simulink model "initial_setup"  (R2012b)
settings: Solver=FixedStepDiscrete  StartTime=0.0  StopTime=inf  FixedStep=sample_time  RelTol=1e-3
InitFcn:
  | init_initial_setup;
values from neighbouring files (symbols this model uses):
  fcut_unwrap = 50    [init_initial_setup.m]
  fcut_velocity = 100    [init_initial_setup.m]
  sample_time = 1/update_freq    (= 0.001)    [init_initial_setup.m]
undefined symbols (not defined in the file or in its folder): A_angle_h, A_angle_k, A_angle_lat, angle_midpoint_h, angle_midpoint_k, angle_midpoint_lat, BOOM_MAX_ENCODER_TICKS, BOOM_PITCH_CAL_VALUE_RAD, BOOM_PITCH_CAL_VALUE_TICKS, BOOM_PITCH_ENCODER_RAD_PER_TICK, BOOM_ROLL_CAL_VALUE_RAD, BOOM_ROLL_CAL_VALUE_TICKS, BOOM_ROLL_ENCODER_RAD_PER_TICK, BOOM_YAW_ENCODER_RAD_PER_TICK, control_start_time, HIP_ABS_ENCODER_RAD_PER_TICK, HIP_INC_ENCODER_RAD_PER_TICK, HIP_INC_MAX_ENCODER_TICKS, k_leg_spring, kd_h_sine_walk, kd_k_sine_walk, kd_lat, kd_sea_position, kd_sea_torque, kd_velocity, kp_h_sine_walk, kp_k_sine_walk, kp_lat, kp_sea_position, kp_sea_torque, kp_velocity, LEFT_HIP_CALIB_POS, LEFT_HIP_CALIB_VAL, LEFT_MOTOR_HIP_DIRECTION, LEG1_LEG_A_CALIB_VAL, LEG1_LEG_A_RAD_PER_CNT, LEG1_LEG_B_CALIB_VAL, LEG1_LEG_B_RAD_PER_CNT, LEG1_MOTOR_A_DIRECTION, LEG1_MOTOR_B_DIRECTION, LEG1_TRAN_A_CALIB_VAL, LEG1_TRAN_A_RAD_PER_CNT, LEG1_TRAN_B_CALIB_VAL, LEG1_TRAN_B_RAD_PER_CNT, LEG2_LEG_A_CALIB_VAL, LEG2_LEG_A_RAD_PER_CNT, LEG2_LEG_B_CALIB_VAL, LEG2_LEG_B_RAD_PER_CNT, LEG2_MOTOR_A_DIRECTION, LEG2_MOTOR_B_DIRECTION, LEG2_TRAN_A_CALIB_VAL, LEG2_TRAN_A_RAD_PER_CNT, LEG2_TRAN_B_CALIB_VAL, LEG2_TRAN_B_RAD_PER_CNT, LEG_A_CALIB_LOC, LEG_B_CALIB_LOC, LEG_MTR_GEAR_RATIO, LEG_MTR_MAX_TORQUE, LEG_MTR_MAX_VELOCITY, MTR_HIP_MAX_CURRENT ... (+10)
libraries: xpcethercatlib x160, simulink x34, dspswit3 x1
(part 1 of 4)
settings Model: xpc_rtwmakecfg_data=_xpcethercatlib_  BufferReuse=off  Creator=wmartin  LastModifiedBy=wmartin
settings DataIOCC: MaxDataPoints=1000000000  SaveFormat=StructureWithTime
settings OptimizationCC: BlockReduction=off  OptimizeBlockIOStorage=off  BufferReuse=off  ExpressionFolding=off  LocalBlockOutputs=off
settings HardwareCC: ProdIntDivRoundTo=Zero  ProdEndianess=LittleEndian  ProdHWDeviceType=Generic->32-bit x86 compatible
settings RTWCC: SystemTargetFile=xpctarget.tlc  TemplateMakefile=xpc_default_tmf  Description=xPC Target  RTWVerbose=off  ProcessScript=xpctarget_make_rtw_hook  RTWCompilerOptimization=On
settings xpcTargetCC: TargetFcnLib=ansi_tfl_table_tmw.mat  CodeReplacementLibrary=XPC_BLAS  ParMdlRefBuildCompliant=on  ConcurrentExecutionCompliant=on  CombineSignalStateStructs=off  GRTInterface=on  RL32LogBufSizeModifier=100000000  xPCTaskExecutionProfile=off  xPCRL32EventNumber=5000  xPCLoadParamSetFile=off  xPCConcurrentTasks=off  xPCEnableSFAnimation=off

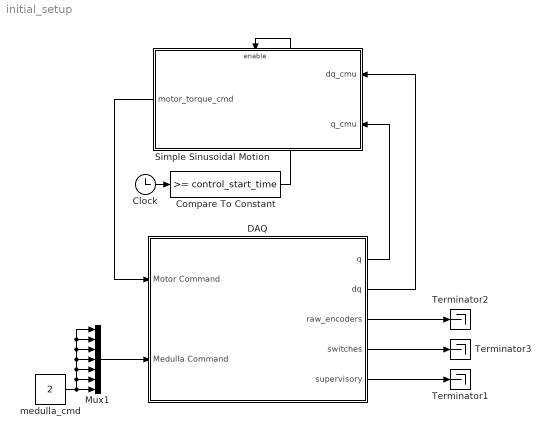
== system initial_setup ==
  Clock : Clock
  Compare To Constant : simulink/Logic and Bit Operations/Compare To Constant  relop=>=  const=control_start_time  OutDataTypeStr=boolean
  DAQ : Subsystem
  Mux1 : Mux  Inputs=7
  Simple Sinusoidal Motion : Subsystem
  Terminator1 : Terminator
  Terminator2 : Terminator
  Terminator3 : Terminator
  medulla_cmd : Constant  Value=2
  wires:
  Mux1/1 -> DAQ/2(Medulla Command)
  DAQ/5(supervisory) -> Terminator1/1
  DAQ/3(raw_encoders) -> Terminator2/1
  DAQ/4(switches) -> Terminator3/1
  Simple Sinusoidal Motion/1(motor_torque_cmd) -> DAQ/1(Motor Command)
  DAQ/1(q) -> Simple Sinusoidal Motion/2(q_cmu)
  DAQ/2(dq) -> Simple Sinusoidal Motion/1(dq_cmu)
  Clock/1 -> Compare To Constant/1
  Compare To Constant/1 -> Simple Sinusoidal Motion/Enable
  medulla_cmd/1 -> Mux1/7, Mux1/1, Mux1/2, Mux1/3, Mux1/4, Mux1/5, Mux1/6

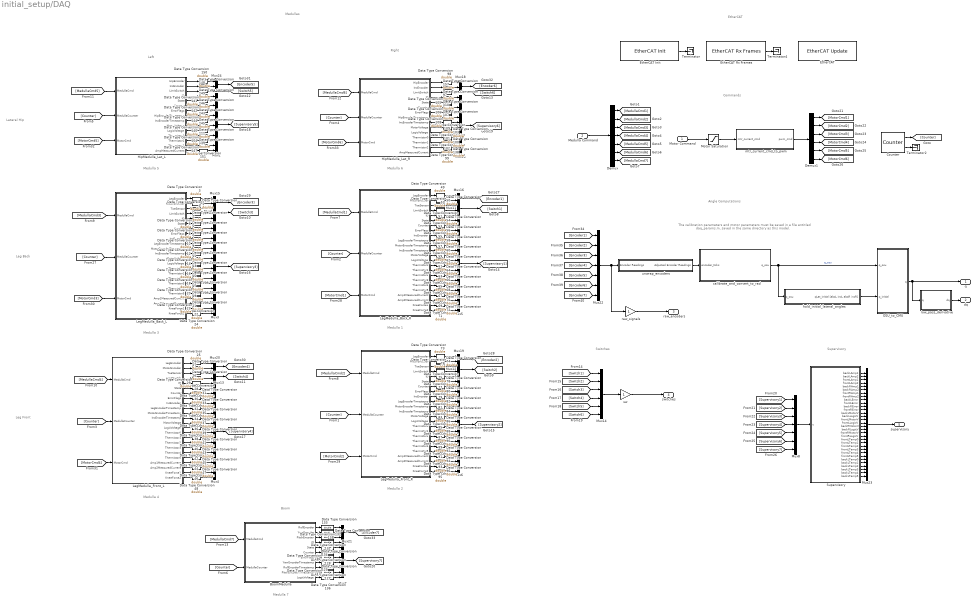
== system initial_setup/DAQ ==
  note: Left
  note: The calibration parameters and motor parameters
      | must be saved in a file entitled daq_params.m, saved in the same directory
      | as this model.
  note: Right
  note: Lateral Hip
  note: Leg Back
  note: Leg Front
  note: Boom
  note: Medullas
  note: EtherCAT
  note: Angle Computations
  note: Commands
  note: Switches
  note: Supervisory
  note: Medulla 1
  note: Medulla 2
  note: Medulla 4
  note: Medulla 3
  note: Medulla 5
  note: Medulla 6
  note: Medulla 7
  Motor Command : Inport
  Medulla Command : Inport  Port=2
  BoomMedulla : Subsystem
  Counter : dspswit3/Counter  Direction=Up  CountEvent=Free running  CounterSize=User defined  MaxCount=65535  InitialCount=0  Output=Count and Hit  HitValue=32  ResetInput=off  SamplesPerFrame=1  Ts=.001  CntDtype=double  HitDtype=Logical
  Data Type Conversion{1..111,127..151,157} (137 alike) : DataTypeConversion  OutDataTypeStr=double
  Demux : Demux  Outputs=7
  Demux1 : Demux  Outputs=6
  EtherCAT : xpcethercatlib/EtherCAT Update   Priority=4  device_id=0  task_id_list=[1]  task_rates=[1]  task_priorities=[1500]
  EtherCAT Init : xpcethercatlib/EtherCAT Init   Priority=0  config_file='atrias_boom.xml'  device_id=0  pci_bus=2  pci_slot=2  enaDC=on  errRptLevel=0  sample_time=-1
  EtherCAT Rx Frames : xpcethercatlib/EtherCAT Rx Frames   Priority=1  device_id=0  sample_time=0
  HipMedulla_Lat_L : Subsystem
  HipMedulla_Lat_R : Subsystem
  LegMedulla_Back_L : Subsystem
  LegMedulla_Back_R : Subsystem
  LegMedulla_Front_L : Subsystem
  LegMedulla_Front_R : Subsystem
  Motor Saturation : Saturate  UpperLimit=60  LowerLimit=-60
  Mux1 : Mux  Inputs=12
  Mux10 : Mux  Inputs=12
  Mux{2,11..13,15..16,18..20,24} (10 alike) : Mux  Inputs=2
  Mux14 : Mux  Inputs=6
  Mux21 : Mux  Inputs=3
  Mux22 : Mux  Inputs=7
  Mux23 : Mux  Inputs=32
  Mux{3..6} (4 alike) : Mux  Inputs=20
  Mux7 : Mux  Inputs=8
  Mux8 : Mux  Inputs=7
  OSU_to_CMU : Subsystem
  Supervisory : MATLAB Function  TreatAsAtomicUnit=on
  Terminator : Terminator
  Terminator2 : Terminator
  Terminator4 : Terminator
  calibrate_and_convert_to_rad : Subsystem
  hold_initial_lateral_angles : Subsystem
  low_pass_derivative : Subsystem
  mtr_current_cmd_to_pwm : Subsystem
  raw_signals : Gain
  sw : Gain
  unwrap_encoders : Subsystem
  q : Outport
  dq : Outport  Port=2
  raw_encoders : Outport  Port=3
  switches : Outport  Port=4
  supervisory : Outport  Port=5
  wires:
  EtherCAT Rx Frames/1 -> Terminator4/1
  OSU_to_CMU/1(q) -> q/1, low_pass_derivative/1(q)
  raw_signals/1 -> raw_encoders/1
  BoomMedulla/11(LogicVoltage) -> Data Type Conversion136/1
  BoomMedulla/10(PitchEncoderTimestamp) -> Data Type Conversion137/1
  BoomMedulla/9(RollEncoderTimestamp) -> Data Type Conversion127/1
  BoomMedulla/8(YawEncoderTimestamp) -> Data Type Conversion129/1
  BoomMedulla/7(ErrorFlags) -> Data Type Conversion130/1
  BoomMedulla/6(Counter) -> Data Type Conversion128/1
  BoomMedulla/5(State) -> Data Type Conversion134/1
  BoomMedulla/4(ID) -> Data Type Conversion135/1
  BoomMedulla/3(PitchEncoder) -> Data Type Conversion131/1
  BoomMedulla/2(YawEncoder) -> Data Type Conversion132/1
  BoomMedulla/1(RollEncoder) -> Data Type Conversion133/1
  Data Type Conversion133/1 -> Mux21/1
  Data Type Conversion132/1 -> Mux21/2
  Data Type Conversion131/1 -> Mux21/3
  Data Type Conversion135/1 -> Mux7/1
  Data Type Conversion134/1 -> Mux7/2
  Data Type Conversion128/1 -> Mux7/3
  Data Type Conversion130/1 -> Mux7/4
  Data Type Conversion129/1 -> Mux7/5
  Data Type Conversion127/1 -> Mux7/6
  Data Type Conversion137/1 -> Mux7/7
  Data Type Conversion136/1 -> Mux7/8
  HipMedulla_Lat_R/15(AmpMeasuredCurrent) -> Data Type Conversion138/1
  HipMedulla_Lat_R/14(Thermistor2) -> Data Type Conversion99/1
  HipMedulla_Lat_R/13(Thermistor1) -> Data Type Conversion100/1
  HipMedulla_Lat_R/12(Thermistor0) -> Data Type Conversion102/1
  HipMedulla_Lat_R/11(LogicVoltage) -> Data Type Conversion103/1
  HipMedulla_Lat_R/10(MotorVoltage) -> Data Type Conversion101/1
  HipMedulla_Lat_R/9(IncEncoderTimestamp) -> Data Type Conversion108/1
  HipMedulla_Lat_R/8(HipEncoderTimestamp) -> Data Type Conversion109/1
  HipMedulla_Lat_R/7(ErrorFlags) -> Data Type Conversion106/1
  HipMedulla_Lat_R/6(Counter) -> Data Type Conversion107/1
  HipMedulla_Lat_R/5(State) -> Data Type Conversion105/1
  HipMedulla_Lat_R/4(ID) -> Data Type Conversion110/1
  HipMedulla_Lat_R/3(LimitSwitch) -> Data Type Conversion157/1
  HipMedulla_Lat_R/2(IncEncoder) -> Data Type Conversion97/1
  HipMedulla_Lat_R/1(HipEncoder) -> Data Type Conversion98/1
  Data Type Conversion98/1 -> Mux18/1
  Data Type Conversion97/1 -> Mux18/2
  Data Type Conversion110/1 -> Mux10/1
  Data Type Conversion105/1 -> Mux10/2
  Data Type Conversion107/1 -> Mux10/3
  Data Type Conversion106/1 -> Mux10/4
  Data Type Conversion109/1 -> Mux10/5
  Data Type Conversion108/1 -> Mux10/6
  Data Type Conversion101/1 -> Mux10/7
  Data Type Conversion103/1 -> Mux10/8
  Data Type Conversion102/1 -> Mux10/9
  Data Type Conversion100/1 -> Mux10/10
  Data Type Conversion99/1 -> Mux10/11
  mtr_current_cmd_to_pwm/1(pwm_cmd) -> Demux1/1
  Data Type Conversion50/1 -> Mux16/2
  Data Type Conversion49/1 -> Mux16/1
  Data Type Conversion48/1 -> Mux4/20
  Data Type Conversion47/1 -> Mux4/19
  Data Type Conversion46/1 -> Mux4/18
  Data Type Conversion45/1 -> Mux4/17
  Data Type Conversion44/1 -> Mux4/16
  Data Type Conversion43/1 -> Mux4/15
  Data Type Conversion42/1 -> Mux4/14
  Data Type Conversion41/1 -> Mux4/13
  Data Type Conversion40/1 -> Mux4/12
  Data Type Conversion39/1 -> Mux4/11
  Data Type Conversion38/1 -> Mux4/10
  Data Type Conversion37/1 -> Mux4/9
  Data Type Conversion36/1 -> Mux4/8
  Data Type Conversion35/1 -> Mux4/7
  Data Type Conversion34/1 -> Mux4/6
  Data Type Conversion33/1 -> Mux4/5
  Data Type Conversion32/1 -> Mux4/4
  Data Type Conversion31/1 -> Mux4/3
  Data Type Conversion30/1 -> Mux4/2
  Data Type Conversion29/1 -> Mux4/1
  Data Type Conversion28/1 -> Mux13/2
  Data Type Conversion27/1 -> Mux13/1
  Data Type Conversion26/1 -> Mux20/2
  Data Type Conversion25/1 -> Mux20/1
  Data Type Conversion24/1 -> Mux3/20
  Data Type Conversion23/1 -> Mux3/19
  Data Type Conversion22/1 -> Mux3/18
  Data Type Conversion21/1 -> Mux3/17
  Data Type Conversion20/1 -> Mux3/16
  Data Type Conversion19/1 -> Mux3/15
  Data Type Conversion18/1 -> Mux3/14
  Data Type Conversion17/1 -> Mux3/13
  Data Type Conversion16/1 -> Mux3/12
  Data Type Conversion15/1 -> Mux3/11
  Data Type Conversion14/1 -> Mux3/10
  Data Type Conversion13/1 -> Mux3/9
  Data Type Conversion12/1 -> Mux3/8
  Data Type Conversion11/1 -> Mux3/7
  Data Type Conversion10/1 -> Mux3/6
  Data Type Conversion9/1 -> Mux3/5
  Data Type Conversion8/1 -> Mux3/4
  Data Type Conversion7/1 -> Mux3/3
  Data Type Conversion6/1 -> Mux3/2
  Data Type Conversion5/1 -> Mux3/1
  Data Type Conversion4/1 -> Mux2/2
  Data Type Conversion2/1 -> Mux2/1
  Data Type Conversion1/1 -> Mux15/2
  Data Type Conversion3/1 -> Mux15/1
  LegMedulla_Back_R/1(LegEncoder) -> Data Type Conversion49/1
  LegMedulla_Back_L/1(LegEncoder) -> Data Type Conversion3/1
  LegMedulla_Back_R/2(MotorEncoder) -> Data Type Conversion50/1
  Motor Saturation/1 -> mtr_current_cmd_to_pwm/1(mtr_current_cmd)
  Motor Command/1 -> Motor Saturation/1
  Data Type Conversion138/1 -> Mux10/12
  Data Type Conversion96/1 -> Mux6/20
  Data Type Conversion95/1 -> Mux6/19
  Data Type Conversion94/1 -> Mux6/18
  Data Type Conversion93/1 -> Mux6/17
  Data Type Conversion92/1 -> Mux6/16
  Data Type Conversion91/1 -> Mux6/15
  Data Type Conversion90/1 -> Mux6/14
  Data Type Conversion89/1 -> Mux6/13
  Data Type Conversion88/1 -> Mux6/12
  Data Type Conversion87/1 -> Mux6/11
  Data Type Conversion86/1 -> Mux6/10
  Data Type Conversion85/1 -> Mux6/9
  Data Type Conversion84/1 -> Mux6/8
  Data Type Conversion83/1 -> Mux6/7
  Data Type Conversion82/1 -> Mux6/6
  Data Type Conversion81/1 -> Mux6/5
  Data Type Conversion80/1 -> Mux6/4
  Data Type Conversion79/1 -> Mux6/3
  Data Type Conversion78/1 -> Mux6/2
  Data Type Conversion77/1 -> Mux6/1
  Data Type Conversion76/1 -> Mux12/2
  Data Type Conversion75/1 -> Mux12/1
  Data Type Conversion74/1 -> Mux19/2
  Data Type Conversion73/1 -> Mux19/1
  Data Type Conversion72/1 -> Mux5/20
  Data Type Conversion71/1 -> Mux5/19
  Data Type Conversion70/1 -> Mux5/18
  Data Type Conversion69/1 -> Mux5/17
  Data Type Conversion68/1 -> Mux5/16
  Data Type Conversion67/1 -> Mux5/15
  Data Type Conversion66/1 -> Mux5/14
  Data Type Conversion65/1 -> Mux5/13
  Data Type Conversion64/1 -> Mux5/12
  Data Type Conversion63/1 -> Mux5/11
  Data Type Conversion62/1 -> Mux5/10
  Data Type Conversion61/1 -> Mux5/9
  Data Type Conversion60/1 -> Mux5/8
  Data Type Conversion59/1 -> Mux5/7
  Data Type Conversion58/1 -> Mux5/6
  Data Type Conversion57/1 -> Mux5/5
  Data Type Conversion56/1 -> Mux5/4
  Data Type Conversion55/1 -> Mux5/3
  Data Type Conversion54/1 -> Mux5/2
  Data Type Conversion53/1 -> Mux5/1
  Data Type Conversion52/1 -> Mux11/2
  Data Type Conversion51/1 -> Mux11/1
  LegMedulla_Front_R/3(ToeSensor) -> Data Type Conversion75/1
  LegMedulla_Front_R/2(MotorEncoder) -> Data Type Conversion74/1
  LegMedulla_Front_R/1(LegEncoder) -> Data Type Conversion73/1
  Counter/2 -> Terminator2/1
  EtherCAT Init/1 -> Terminator/1
  Medulla Command/1 -> Demux/1
  LegMedulla_Front_R/24(KneeForce2) -> Data Type Conversion96/1
  LegMedulla_Back_R/24(KneeForce2) -> Data Type Conversion72/1
  LegMedulla_Front_R/23(KneeForce1) -> Data Type Conversion95/1
  LegMedulla_Front_R/22(Amp2MeasuredCurrent) -> Data Type Conversion94/1
  LegMedulla_Front_R/21(Amp1MeasuredCurrent) -> Data Type Conversion93/1
  LegMedulla_Front_R/20(Thermistor5) -> Data Type Conversion92/1
  LegMedulla_Front_R/19(Thermistor4) -> Data Type Conversion91/1
  LegMedulla_Front_R/18(Thermistor3) -> Data Type Conversion90/1
  LegMedulla_Front_R/17(Thermistor2) -> Data Type Conversion89/1
  LegMedulla_Front_R/16(Thermistor1) -> Data Type Conversion88/1
  LegMedulla_Front_R/15(Thermistor0) -> Data Type Conversion87/1
  LegMedulla_Front_R/14(LogicVoltage) -> Data Type Conversion86/1
  LegMedulla_Front_R/13(MotorVoltage) -> Data Type Conversion85/1
  LegMedulla_Front_R/12(IncEncoderTimestamp) -> Data Type Conversion84/1
  LegMedulla_Front_R/11(MotorEncoderTimestamp) -> Data Type Conversion83/1
  LegMedulla_Front_R/10(LegEncoderTimestamp) -> Data Type Conversion82/1
  LegMedulla_Front_R/9(IncEncoder) -> Data Type Conversion81/1
  LegMedulla_Front_R/8(ErrorFlags) -> Data Type Conversion80/1
  LegMedulla_Front_R/7(Counter) -> Data Type Conversion79/1
  LegMedulla_Front_R/6(State) -> Data Type Conversion78/1
  LegMedulla_Front_R/5(ID) -> Data Type Conversion77/1
  LegMedulla_Front_R/4(LimitSwitch) -> Data Type Conversion76/1
  LegMedulla_Back_R/23(KneeForce1) -> Data Type Conversion71/1
  LegMedulla_Back_R/22(Amp2MeasuredCurrent) -> Data Type Conversion70/1
  LegMedulla_Back_R/21(Amp1MeasuredCurrent) -> Data Type Conversion69/1
  LegMedulla_Back_R/20(Thermistor5) -> Data Type Conversion68/1
  LegMedulla_Back_R/19(Thermistor4) -> Data Type Conversion67/1
  LegMedulla_Back_R/18(Thermistor3) -> Data Type Conversion66/1
  LegMedulla_Back_R/17(Thermistor2) -> Data Type Conversion65/1
  LegMedulla_Back_R/16(Thermistor1) -> Data Type Conversion64/1
  LegMedulla_Back_R/15(Thermistor0) -> Data Type Conversion63/1
  LegMedulla_Back_R/14(LogicVoltage) -> Data Type Conversion62/1
  LegMedulla_Back_R/13(MotorVoltage) -> Data Type Conversion61/1
  LegMedulla_Back_R/12(IncEncoderTimestamp) -> Data Type Conversion60/1
  LegMedulla_Back_R/11(MotorEncoderTimestamp) -> Data Type Conversion59/1
  LegMedulla_Back_R/10(LegEncoderTimestamp) -> Data Type Conversion58/1
  LegMedulla_Back_R/9(IncEncoder) -> Data Type Conversion57/1
  LegMedulla_Back_R/8(ErrorFlags) -> Data Type Conversion56/1
  LegMedulla_Back_R/7(Counter) -> Data Type Conversion55/1
  LegMedulla_Back_R/6(State) -> Data Type Conversion54/1
  LegMedulla_Back_R/5(ID) -> Data Type Conversion53/1
  LegMedulla_Back_R/4(LimitSwitch) -> Data Type Conversion52/1
  LegMedulla_Back_R/3(ToeSensor) -> Data Type Conversion51/1
  LegMedulla_Front_L/24(KneeForce2) -> Data Type Conversion48/1
  LegMedulla_Back_L/24(KneeForce2) -> Data Type Conversion24/1
  LegMedulla_Front_L/23(KneeForce1) -> Data Type Conversion47/1
  LegMedulla_Front_L/22(Amp2MeasuredCurrent) -> Data Type Conversion46/1
  LegMedulla_Front_L/21(Amp1MeasuredCurrent) -> Data Type Conversion45/1
  LegMedulla_Front_L/20(Thermistor5) -> Data Type Conversion44/1
  LegMedulla_Front_L/19(Thermistor4) -> Data Type Conversion43/1
  LegMedulla_Front_L/18(Thermistor3) -> Data Type Conversion42/1
  LegMedulla_Front_L/17(Thermistor2) -> Data Type Conversion41/1
  LegMedulla_Front_L/16(Thermistor1) -> Data Type Conversion40/1
  LegMedulla_Front_L/15(Thermistor0) -> Data Type Conversion39/1
  LegMedulla_Front_L/14(LogicVoltage) -> Data Type Conversion38/1
  LegMedulla_Front_L/13(MotorVoltage) -> Data Type Conversion37/1
  LegMedulla_Front_L/12(IncEncoderTimestamp) -> Data Type Conversion36/1
  LegMedulla_Front_L/11(MotorEncoderTimestamp) -> Data Type Conversion35/1
  LegMedulla_Front_L/10(LegEncoderTimestamp) -> Data Type Conversion34/1
  LegMedulla_Front_L/9(IncEncoder) -> Data Type Conversion33/1
  LegMedulla_Front_L/8(ErrorFlags) -> Data Type Conversion32/1
  LegMedulla_Front_L/7(Counter) -> Data Type Conversion31/1
  LegMedulla_Front_L/6(State) -> Data Type Conversion30/1
  LegMedulla_Front_L/5(ID) -> Data Type Conversion29/1
  LegMedulla_Front_L/4(LimitSwitch) -> Data Type Conversion28/1
  LegMedulla_Front_L/3(ToeSensor) -> Data Type Conversion27/1
  LegMedulla_Front_L/2(MotorEncoder) -> Data Type Conversion26/1
  LegMedulla_Front_L/1(LegEncoder) -> Data Type Conversion25/1
  LegMedulla_Back_L/23(KneeForce1) -> Data Type Conversion23/1
  LegMedulla_Back_L/22(Amp2MeasuredCurrent) -> Data Type Conversion22/1
  LegMedulla_Back_L/21(Amp1MeasuredCurrent) -> Data Type Conversion21/1
  LegMedulla_Back_L/20(Thermistor5) -> Data Type Conversion20/1
  LegMedulla_Back_L/19(Thermistor4) -> Data Type Conversion19/1
  LegMedulla_Back_L/18(Thermistor3) -> Data Type Conversion18/1
  LegMedulla_Back_L/17(Thermistor2) -> Data Type Conversion17/1
  LegMedulla_Back_L/16(Thermistor1) -> Data Type Conversion16/1
  LegMedulla_Back_L/15(Thermistor0) -> Data Type Conversion15/1
  LegMedulla_Back_L/14(LogicVoltage) -> Data Type Conversion14/1
  LegMedulla_Back_L/13(MotorVoltage) -> Data Type Conversion13/1
  LegMedulla_Back_L/12(IncEncoderTimestamp) -> Data Type Conversion12/1
  LegMedulla_Back_L/11(MotorEncoderTimestamp) -> Data Type Conversion11/1
  LegMedulla_Back_L/10(LegEncoderTimestamp) -> Data Type Conversion10/1
  LegMedulla_Back_L/9(IncEncoder) -> Data Type Conversion9/1
  LegMedulla_Back_L/8(ErrorFlags) -> Data Type Conversion8/1
  LegMedulla_Back_L/7(Counter) -> Data Type Conversion7/1
  LegMedulla_Back_L/6(State) -> Data Type Conversion6/1
  LegMedulla_Back_L/5(ID) -> Data Type Conversion5/1
  LegMedulla_Back_L/4(LimitSwitch) -> Data Type Conversion4/1
  LegMedulla_Back_L/3(ToeSensor) -> Data Type Conversion2/1
  LegMedulla_Back_L/2(MotorEncoder) -> Data Type Conversion1/1
  Counter/1 -> [Counter]
  [Counter] -> LegMedulla_Back_L/2(MedullaCounter)
  [Counter] -> LegMedulla_Front_L/2(MedullaCounter)
  [Counter] -> LegMedulla_Back_R/2(MedullaCounter)
  [Counter] -> LegMedulla_Front_R/2(MedullaCounter)
  [Counter] -> HipMedulla_Lat_R/2(MedullaCounter)
  [Counter] -> HipMedulla_Lat_L/2(MedullaCounter)
  [Counter] -> BoomMedulla/2(MedullaCounter)
  Demux/2 -> [MedullaCmd2]
  Demux/1 -> [MedullaCmd1]
  Demux/3 -> [MedullaCmd3]
  Demux/4 -> [MedullaCmd4]
  Demux/5 -> [MedullaCmd5]
  Demux/6 -> [MedullaCmd6]
  Demux/7 -> [MedullaCmd7]
  [MedullaCmd3] -> LegMedulla_Back_L/1(MedullaCmd)
  [MedullaCmd4] -> LegMedulla_Front_L/1(MedullaCmd)
  [MedullaCmd1] -> LegMedulla_Back_R/1(MedullaCmd)
  [MedullaCmd2] -> LegMedulla_Front_R/1(MedullaCmd)
  [MedullaCmd6] -> HipMedulla_Lat_R/1(MedullaCmd)
  [MedullaCmd7] -> BoomMedulla/1(MedullaCmd)
  [MedullaCmd5] -> HipMedulla_Lat_L/1(MedullaCmd)
  Data Type Conversion157/1 -> [Switch6]
  [Switch1] -> Mux14/1
  [Switch2] -> Mux14/2
  [Switch3] -> Mux14/3
  [Switch4] -> Mux14/4
  [Switch5] -> Mux14/5
  [Switch6] -> Mux14/6
  sw/1 -> switches/1
  low_pass_derivative/1(dq) -> dq/1
  calibrate_and_convert_to_rad/1(q_osu) -> hold_initial_lateral_angles/1(q_osu), OSU_to_CMU/1(q_osu)  "q_osu"
  hold_initial_lateral_angles/1(qLat_initial [absL incL absR incR]) -> OSU_to_CMU/2(q_initial)
  unwrap_encoders/1(Adjusted Encoder Readings) -> calibrate_and_convert_to_rad/1(encoder_ticks)
  [MotorCmd3] -> LegMedulla_Back_L/3(MotorCmd)
  [MotorCmd4] -> LegMedulla_Front_L/3(MotorCmd)
  [MotorCmd1] -> LegMedulla_Back_R/3(MotorCmd)
  [MotorCmd2] -> LegMedulla_Front_R/3(MotorCmd)
  [MotorCmd6] -> HipMedulla_Lat_R/3(MotorCmd)
  [MotorCmd5] -> HipMedulla_Lat_L/3(MotorCmd)
  Demux1/1 -> [MotorCmd1]
  Demux1/2 -> [MotorCmd2]
  Demux1/3 -> [MotorCmd3]
  Demux1/4 -> [MotorCmd4]
  Demux1/5 -> [MotorCmd5]
  Demux1/6 -> [MotorCmd6]
  Mux2/1 -> [Switch3]
  Mux3/1 -> [Supervisory3]
  Mux4/1 -> [Supervisory4]
  Mux5/1 -> [Supervisory1]
  Mux6/1 -> [Supervisory2]
  Mux7/1 -> [Supervisory7]
  [Supervisory1] -> Mux8/1
  [Supervisory2] -> Mux8/2
  [Supervisory3] -> Mux8/3
  [Supervisory4] -> Mux8/4
  [Supervisory5] -> Mux8/5
  [Supervisory6] -> Mux8/6
  [Supervisory7] -> Mux8/7
  Mux8/1 -> Supervisory/1(u)
  Mux10/1 -> [Supervisory6]
  Mux11/1 -> [Switch1]
  Mux12/1 -> [Switch2]
  Mux13/1 -> [Switch4]
  Mux14/1 -> sw/1
  Mux15/1 -> [Encoder3]
  Mux16/1 -> [Encoder1]
  Mux18/1 -> [Encoder6]
  Mux19/1 -> [Encoder2]
  Mux20/1 -> [Encoder4]
  Mux21/1 -> [Encoder7]
  [Encoder7] -> Mux22/7
  [Encoder6] -> Mux22/6
  [Encoder5] -> Mux22/5
  [Encoder4] -> Mux22/4
  [Encoder3] -> Mux22/3
  [Encoder2] -> Mux22/2
  [Encoder1] -> Mux22/1
  Mux22/1 -> raw_signals/1, unwrap_encoders/1(Encoder Readings)
  Supervisory/1(backLAmp1) -> Mux23/1
  Supervisory/2(backLAmp2) -> Mux23/2
  Supervisory/3(frontLAmp1) -> Mux23/3
  Supervisory/4(frontLAmp2) -> Mux23/4
  Supervisory/5(backRAmp1) -> Mux23/5
  Supervisory/6(backRAmp2) -> Mux23/6
  Supervisory/7(frontRAmp1) -> Mux23/7
  Supervisory/9(backLError) -> Mux23/9
  Supervisory/8(frontRAmp2) -> Mux23/8
  Supervisory/10(frontLError) -> Mux23/10
  Supervisory/11(backRError) -> Mux23/11
  Supervisory/12(frontRError) -> Mux23/12
  Supervisory/13(backLMotorV) -> Mux23/13
  Supervisory/14(backLLogicV) -> Mux23/14
  Supervisory/15(frontLMotorV) -> Mux23/15
  Supervisory/16(frontLLogicV) -> Mux23/16
  Supervisory/17(backRMotorV) -> Mux23/17
  Supervisory/18(backRLogicV) -> Mux23/18
  Supervisory/19(frontRMotorV) -> Mux23/19
  Supervisory/20(frontRLogicV) -> Mux23/20
  Mux23/1 -> supervisory/1
  HipMedulla_Lat_L/15(AmpMeasuredCurrent) -> Data Type Conversion147/1
  HipMedulla_Lat_L/14(Thermistor2) -> Data Type Conversion151/1
  HipMedulla_Lat_L/13(Thermistor1) -> Data Type Conversion104/1
  HipMedulla_Lat_L/12(Thermistor0) -> Data Type Conversion139/1
  HipMedulla_Lat_L/11(LogicVoltage) -> Data Type Conversion140/1
  HipMedulla_Lat_L/10(MotorVoltage) -> Data Type Conversion111/1
  HipMedulla_Lat_L/9(IncEncoderTimestamp) -> Data Type Conversion144/1
  HipMedulla_Lat_L/8(HipEncoderTimestamp) -> Data Type Conversion145/1
  HipMedulla_Lat_L/7(ErrorFlags) -> Data Type Conversion142/1
  HipMedulla_Lat_L/6(Counter) -> Data Type Conversion143/1
  HipMedulla_Lat_L/5(State) -> Data Type Conversion141/1
  HipMedulla_Lat_L/4(ID) -> Data Type Conversion146/1
  HipMedulla_Lat_L/3(LimitSwitch) -> Data Type Conversion148/1
  HipMedulla_Lat_L/2(IncEncoder) -> Data Type Conversion149/1
  HipMedulla_Lat_L/1(HipEncoder) -> Data Type Conversion150/1
  Data Type Conversion150/1 -> Mux24/1
  Data Type Conversion149/1 -> Mux24/2
  Data Type Conversion146/1 -> Mux1/1
  Data Type Conversion141/1 -> Mux1/2
  Data Type Conversion143/1 -> Mux1/3
  Data Type Conversion142/1 -> Mux1/4
  Data Type Conversion145/1 -> Mux1/5
  Data Type Conversion144/1 -> Mux1/6
  Data Type Conversion111/1 -> Mux1/7
  Data Type Conversion140/1 -> Mux1/8
  Data Type Conversion139/1 -> Mux1/9
  Data Type Conversion104/1 -> Mux1/10
  Data Type Conversion151/1 -> Mux1/11
  Data Type Conversion147/1 -> Mux1/12
  Data Type Conversion148/1 -> [Switch5]
  Mux1/1 -> [Supervisory5]
  Mux24/1 -> [Encoder5]
  Supervisory/21(frontLTemp0) -> Mux23/21
  Supervisory/22(frontLTemp1) -> Mux23/22
  Supervisory/23(frontLTemp2) -> Mux23/23
  Supervisory/24(frontLTemp3) -> Mux23/24
  Supervisory/25(frontLTemp4) -> Mux23/25
  Supervisory/26(frontLTemp5) -> Mux23/26
  Supervisory/28(backLTemp1) -> Mux23/28
  Supervisory/27(backLTemp0) -> Mux23/27
  Supervisory/29(backLTemp2) -> Mux23/29
  Supervisory/30(backLTemp3) -> Mux23/30
  Supervisory/31(backLTemp4) -> Mux23/31
  Supervisory/32(backLTemp5) -> Mux23/32

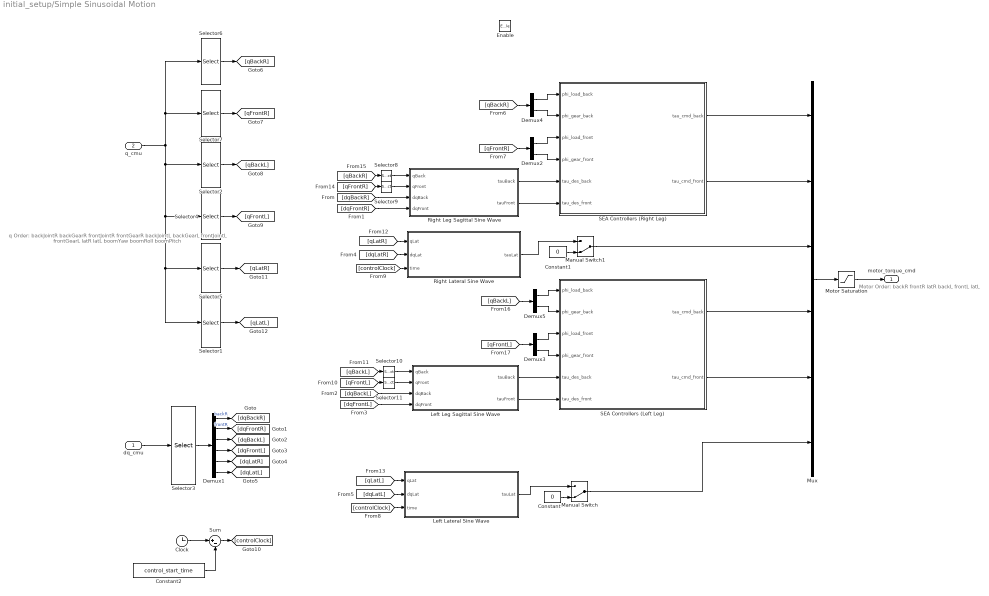
== system initial_setup/Simple Sinusoidal Motion ==
  note: q Order:
      |
      | backJointR
      | backGearR
      | frontJointR
      | frontGearR
      |
      | backJointL
      | backGearL
      | frontJointL
      | frontGearL
      |
      | latR
      | latL
      |
      | boomYaw
      | boomRoll
      | boomPitch
  note: Motor Order:
      |
      | backR
      | frontR
      | latR
      | backL
      | frontL
      | latL
  dq_cmu : Inport
  q_cmu : Inport  Port=2
  Enable : EnablePort  StatesWhenEnabling=reset
  Clock : Clock
  Constant : Constant  Value=0
  Constant1 : Constant  Value=0
  Constant2 : Constant  Value=control_start_time
  Demux1 : Demux  Outputs=6
  Demux{2..5} (4 alike) : Demux  Outputs=2
  Left Lateral Sine Wave : Subsystem
  Left Leg Sagittal Sine Wave : Subsystem
  Manual Switch : ManualSwitch  CurrentSetting=0
  Manual Switch1 : ManualSwitch  CurrentSetting=0
  Motor Saturation : Saturate  UpperLimit=6  LowerLimit=-6
  Mux : Mux  Inputs=6
  Right Lateral Sine Wave : Subsystem
  Right Leg Sagittal Sine Wave : Subsystem
  SEA Controllers (Left Leg) : Subsystem
  SEA Controllers (Right Leg) : Subsystem
  Selector1 : Selector  InputPortWidth=13  IndexOptions=Index vector (dialog)  Indices=[10]  OutputSizes=1
  Selector{8..11} (4 alike) : Selector  InputPortWidth=2  IndexOptions=Index vector (dialog)  Indices=[2]  OutputSizes=1
  Selector2 : Selector  InputPortWidth=13  IndexOptions=Index vector (dialog)  Indices=[5 6]  OutputSizes=1
  Selector3 : Selector  InputPortWidth=13  IndexOptions=Index vector (dialog)  Indices=[2 4 6 8 9 10]  OutputSizes=1
  Selector4 : Selector  InputPortWidth=13  IndexOptions=Index vector (dialog)  Indices=[7 8]  OutputSizes=1
  Selector5 : Selector  InputPortWidth=13  IndexOptions=Index vector (dialog)  Indices=[9]  OutputSizes=1
  Selector6 : Selector  InputPortWidth=13  IndexOptions=Index vector (dialog)  Indices=[1 2]  OutputSizes=1
  Selector7 : Selector  InputPortWidth=13  IndexOptions=Index vector (dialog)  Indices=[3 4]  OutputSizes=1
  Sum : Sum  Inputs=|+-
  motor_torque_cmd : Outport  OutputWhenDisabled=reset  InitialOutput=[0 0 0 0 0 0]
  wires:
  Mux/1 -> Motor Saturation/1
  Motor Saturation/1 -> motor_torque_cmd/1
  dq_cmu/1 -> Selector3/1
  Selector3/1 -> Demux1/1
  Right Lateral Sine Wave/1(tauLat) -> Manual Switch1/1
  Left Lateral Sine Wave/1(tauLat) -> Manual Switch/1
  Manual Switch1/1 -> Mux/3
  Manual Switch/1 -> Mux/6
  Constant/1 -> Manual Switch/2
  Constant1/1 -> Manual Switch1/2
  Clock/1 -> Sum/1
  Constant2/1 -> Sum/2
  [qBackR] -> Demux4/1
  [qFrontR] -> Demux2/1
  Demux2/2 -> SEA Controllers (Right Leg)/4(phi_gear_front)
  Selector5/1 -> [qLatR]
  Selector1/1 -> [qLatL]
  Demux1/1 -> [dqBackR]  "backR"
  [dqBackR] -> Right Leg Sagittal Sine Wave/3(dqBack)
  [dqFrontR] -> Right Leg Sagittal Sine Wave/4(dqFront)
  Demux1/2 -> [dqFrontR]  "frontR"
  Demux1/3 -> [dqBackL]
  Demux1/4 -> [dqFrontL]
  [dqBackL] -> Left Leg Sagittal Sine Wave/3(dqBack)
  [dqFrontL] -> Left Leg Sagittal Sine Wave/4(dqFront)
  Demux1/5 -> [dqLatR]
  Demux1/6 -> [dqLatL]
  [dqLatR] -> Right Lateral Sine Wave/2(dqLat)
  [dqLatL] -> Left Lateral Sine Wave/2(dqLat)
  Selector6/1 -> [qBackR]
  Selector7/1 -> [qFrontR]
  Selector2/1 -> [qBackL]
  Selector4/1 -> [qFrontL]
  Sum/1 -> [controlClock]
  [controlClock] -> Left Lateral Sine Wave/3(time)
  [controlClock] -> Right Lateral Sine Wave/3(time)
  q_cmu/1 -> Selector1/1, Selector5/1, Selector4/1, Selector2/1, Selector7/1, Selector6/1
  [qLatL] -> Left Lateral Sine Wave/1(qLat)
  [qLatR] -> Right Lateral Sine Wave/1(qLat)
  Right Leg Sagittal Sine Wave/1(tauBack) -> SEA Controllers (Right Leg)/5(tau_des_back)
  Right Leg Sagittal Sine Wave/2(tauFront) -> SEA Controllers (Right Leg)/6(tau_des_front)
  Demux2/1 -> SEA Controllers (Right Leg)/3(phi_load_front)
  SEA Controllers (Right Leg)/1(tau_cmd_back) -> Mux/1
  SEA Controllers (Right Leg)/2(tau_cmd_front) -> Mux/2
  [qBackR] -> Selector8/1
  Selector8/1 -> Right Leg Sagittal Sine Wave/1(qBack)
  [qFrontR] -> Selector9/1
  Selector9/1 -> Right Leg Sagittal Sine Wave/2(qFront)
  Demux4/1 -> SEA Controllers (Right Leg)/1(phi_load_back)
  Demux4/2 -> SEA Controllers (Right Leg)/2(phi_gear_back)
  Selector10/1 -> Left Leg Sagittal Sine Wave/1(qBack)
  Selector11/1 -> Left Leg Sagittal Sine Wave/2(qFront)
  [qBackL] -> Selector10/1
  [qFrontL] -> Selector11/1
  SEA Controllers (Left Leg)/1(tau_cmd_back) -> Mux/4
  SEA Controllers (Left Leg)/2(tau_cmd_front) -> Mux/5
  Left Leg Sagittal Sine Wave/1(tauBack) -> SEA Controllers (Left Leg)/5(tau_des_back)
  Left Leg Sagittal Sine Wave/2(tauFront) -> SEA Controllers (Left Leg)/6(tau_des_front)
  [qBackL] -> Demux5/1
  [qFrontL] -> Demux3/1
  Demux3/2 -> SEA Controllers (Left Leg)/4(phi_gear_front)
  Demux3/1 -> SEA Controllers (Left Leg)/3(phi_load_front)
  Demux5/1 -> SEA Controllers (Left Leg)/1(phi_load_back)
  Demux5/2 -> SEA Controllers (Left Leg)/2(phi_gear_back)

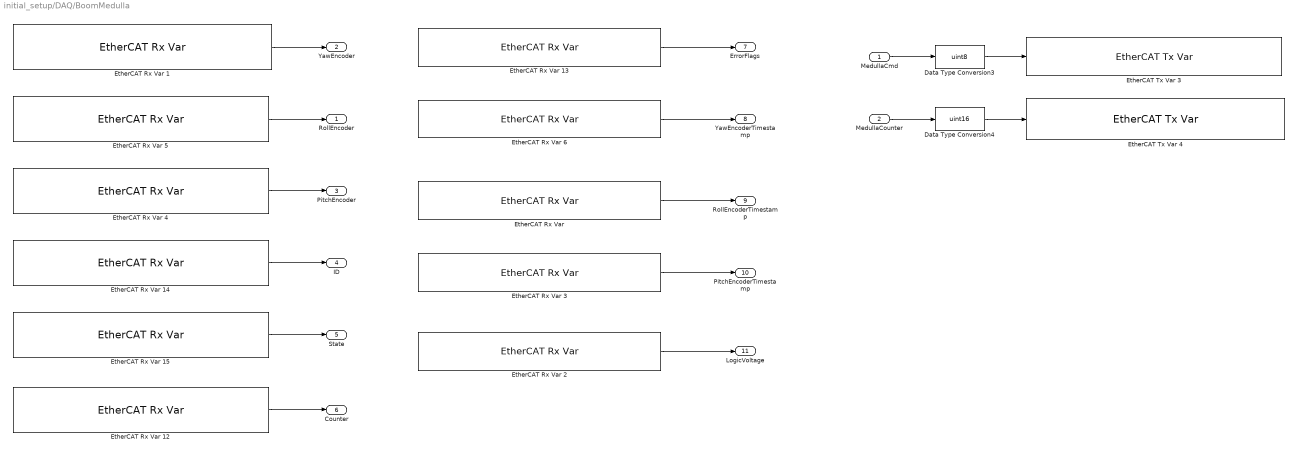
== system initial_setup/DAQ/BoomMedulla ==
  MedullaCmd : Inport
  MedullaCounter : Inport  Port=2
  Data Type Conversion3 : DataTypeConversion  OutDataTypeStr=uint8
  Data Type Conversion4 : DataTypeConversion  OutDataTypeStr=uint16
  "EtherCAT Rx Var " : xpcethercatlib/EtherCAT Rx Var   Priority=2  sig_name=Box 7 (ATRIAS 2.1 Boom (Medulla 1.5)).X Encoder.Timestamp  sig_offset=2464  sig_type=uint16  type_size=16  sig_dim=1  device_id=0  sample_time=0.001000
  EtherCAT Rx Var 1 : xpcethercatlib/EtherCAT Rx Var   Priority=2  sig_name=Box 7 (ATRIAS 2.1 Boom (Medulla 1.5)).Z Encoder.Encoder  sig_offset=2528  sig_type=uint32  type_size=32  sig_dim=1  device_id=0  sample_time=0.001000
  EtherCAT Rx Var 12 : xpcethercatlib/EtherCAT Rx Var   Priority=2  sig_name=Box 7 (ATRIAS 2.1 Boom (Medulla 1.5)).uController Status.Counter  sig_offset=2416  sig_type=uint8  type_size=8  sig_dim=1  device_id=0  sample_time=0.001000
  EtherCAT Rx Var 13 : xpcethercatlib/EtherCAT Rx Var   Priority=2  sig_name=Box 7 (ATRIAS 2.1 Boom (Medulla 1.5)).uController Status.Error Flags  sig_offset=2424  sig_type=uint8  type_size=8  sig_dim=1  device_id=0  sample_time=0.001000
  EtherCAT Rx Var 14 : xpcethercatlib/EtherCAT Rx Var   Priority=2  sig_name=Box 7 (ATRIAS 2.1 Boom (Medulla 1.5)).uController Status.ID  sig_offset=2400  sig_type=uint8  type_size=8  sig_dim=1  device_id=0  sample_time=0.001000
  EtherCAT Rx Var 15 : xpcethercatlib/EtherCAT Rx Var   Priority=2  sig_name=Box 7 (ATRIAS 2.1 Boom (Medulla 1.5)).uController Status.State  sig_offset=2408  sig_type=uint8  type_size=8  sig_dim=1  device_id=0  sample_time=0.001000
  EtherCAT Rx Var 2 : xpcethercatlib/EtherCAT Rx Var   Priority=2  sig_name=Box 7 (ATRIAS 2.1 Boom (Medulla 1.5)).Power.Logic Voltage  sig_offset=2576  sig_type=uint16  type_size=16  sig_dim=1  device_id=0  sample_time=0.001000
  EtherCAT Rx Var 3 : xpcethercatlib/EtherCAT Rx Var   Priority=2  sig_name=Box 7 (ATRIAS 2.1 Boom (Medulla 1.5)).Pitch Encoder.Timestamp  sig_offset=2512  sig_type=uint16  type_size=16  sig_dim=1  device_id=0  sample_time=0.001000
  EtherCAT Rx Var 4 : xpcethercatlib/EtherCAT Rx Var   Priority=2  sig_name=Box 7 (ATRIAS 2.1 Boom (Medulla 1.5)).Pitch Encoder.Encoder  sig_offset=2480  sig_type=uint32  type_size=32  sig_dim=1  device_id=0  sample_time=0.001000
  EtherCAT Rx Var 5 : xpcethercatlib/EtherCAT Rx Var   Priority=2  sig_name=Box 7 (ATRIAS 2.1 Boom (Medulla 1.5)).X Encoder.Encoder  sig_offset=2432  sig_type=uint32  type_size=32  sig_dim=1  device_id=0  sample_time=0.001000
  EtherCAT Rx Var 6 : xpcethercatlib/EtherCAT Rx Var   Priority=2  sig_name=Box 7 (ATRIAS 2.1 Boom (Medulla 1.5)).Z Encoder.Timestamp  sig_offset=2560  sig_type=uint16  type_size=16  sig_dim=1  device_id=0  sample_time=0.001000
  EtherCAT Tx Var 3 : xpcethercatlib/EtherCAT Tx Var   Priority=3  sig_name=Box 7 (ATRIAS 2.1 Boom (Medulla 1.5)).uControllerInput.Command  sig_offset=2400  sig_type=uint8  type_size=8  sig_dim=1  device_id=0  sample_time=0.001000
  EtherCAT Tx Var 4 : xpcethercatlib/EtherCAT Tx Var   Priority=3  sig_name=Box 7 (ATRIAS 2.1 Boom (Medulla 1.5)).uControllerInput.Counter  sig_offset=2408  sig_type=uint16  type_size=16  sig_dim=1  device_id=0  sample_time=0.001000
  RollEncoder : Outport
  YawEncoder : Outport  Port=2
  PitchEncoder : Outport  Port=3
  ID : Outport  Port=4
  State : Outport  Port=5
  Counter : Outport  Port=6
  ErrorFlags : Outport  Port=7
  YawEncoderTimestamp : Outport  Port=8
  RollEncoderTimestamp : Outport  Port=9
  PitchEncoderTimestamp : Outport  Port=10
  LogicVoltage : Outport  Port=11
  wires:
  EtherCAT Rx Var 2/1 -> LogicVoltage/1
  EtherCAT Rx Var 3/1 -> PitchEncoderTimestamp/1
  "EtherCAT Rx Var "/1 -> RollEncoderTimestamp/1
  EtherCAT Rx Var 6/1 -> YawEncoderTimestamp/1
  EtherCAT Rx Var 13/1 -> ErrorFlags/1
  EtherCAT Rx Var 12/1 -> Counter/1
  EtherCAT Rx Var 15/1 -> State/1
  EtherCAT Rx Var 14/1 -> ID/1
  EtherCAT Rx Var 4/1 -> PitchEncoder/1
  EtherCAT Rx Var 5/1 -> RollEncoder/1
  EtherCAT Rx Var 1/1 -> YawEncoder/1
  MedullaCounter/1 -> Data Type Conversion4/1
  MedullaCmd/1 -> Data Type Conversion3/1
  Data Type Conversion4/1 -> EtherCAT Tx Var 4/1
  Data Type Conversion3/1 -> EtherCAT Tx Var 3/1

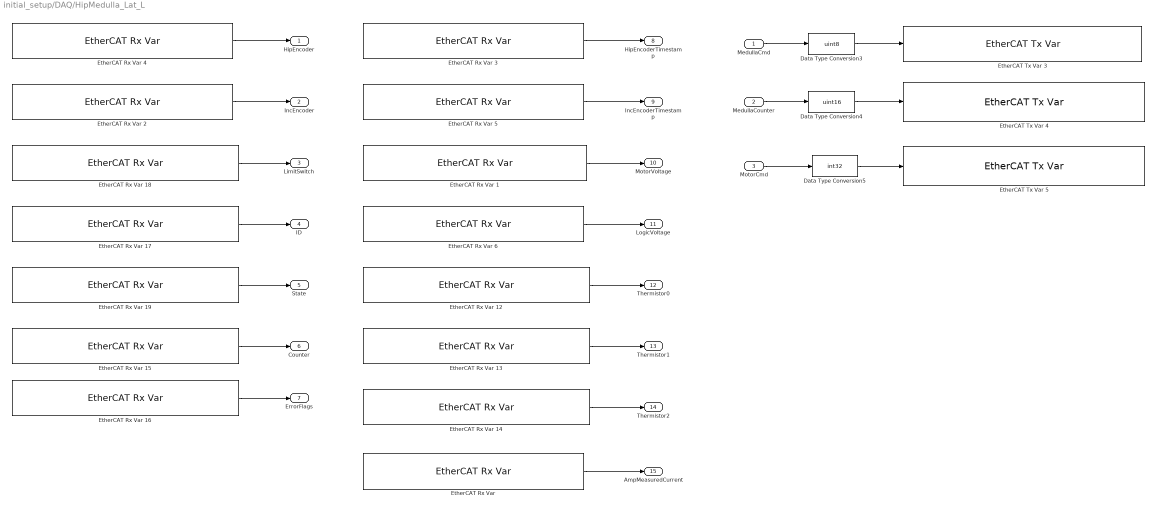
== system initial_setup/DAQ/HipMedulla_Lat_L ==
  MedullaCmd : Inport
  MedullaCounter : Inport  Port=2
  MotorCmd : Inport  Port=3
  Data Type Conversion3 : DataTypeConversion  OutDataTypeStr=uint8
  Data Type Conversion4 : DataTypeConversion  OutDataTypeStr=uint16
  Data Type Conversion5 : DataTypeConversion  OutDataTypeStr=int32
  "EtherCAT Rx Var " : xpcethercatlib/EtherCAT Rx Var   Priority=2  sig_name=Box 5 (ATRIAS 2.1 Hip (Medulla 1.5)).Measured Current.Amp Measured Current  sig_offset=2136  sig_type=int16  type_size=16  sig_dim=1  device_id=0  sample_time=0.001000
  EtherCAT Rx Var 1 : xpcethercatlib/EtherCAT Rx Var   Priority=2  sig_name=Box 5 (ATRIAS 2.1 Hip (Medulla 1.5)).Power.Motor Voltage  sig_offset=2056  sig_type=uint16  type_size=16  sig_dim=1  device_id=0  sample_time=0.001000
  EtherCAT Rx Var 12 : xpcethercatlib/EtherCAT Rx Var   Priority=2  sig_name=Box 5 (ATRIAS 2.1 Hip (Medulla 1.5)).Thermistors.Thermistor 0  sig_offset=2088  sig_type=uint16  type_size=16  sig_dim=1  device_id=0  sample_time=0.001000
  EtherCAT Rx Var 13 : xpcethercatlib/EtherCAT Rx Var   Priority=2  sig_name=Box 5 (ATRIAS 2.1 Hip (Medulla 1.5)).Thermistors.Thermistor 1  sig_offset=2104  sig_type=uint16  type_size=16  sig_dim=1  device_id=0  sample_time=0.001000
  EtherCAT Rx Var 14 : xpcethercatlib/EtherCAT Rx Var   Priority=2  sig_name=Box 5 (ATRIAS 2.1 Hip (Medulla 1.5)).Thermistors.Thermistor 2  sig_offset=2120  sig_type=uint16  type_size=16  sig_dim=1  device_id=0  sample_time=0.001000
  EtherCAT Rx Var 15 : xpcethercatlib/EtherCAT Rx Var   Priority=2  sig_name=Box 5 (ATRIAS 2.1 Hip (Medulla 1.5)).uController Status.Counter  sig_offset=1984  sig_type=uint8  type_size=8  sig_dim=1  device_id=0  sample_time=0.001000
  EtherCAT Rx Var 16 : xpcethercatlib/EtherCAT Rx Var   Priority=2  sig_name=Box 5 (ATRIAS 2.1 Hip (Medulla 1.5)).uController Status.Error Flags  sig_offset=1992  sig_type=uint8  type_size=8  sig_dim=1  device_id=0  sample_time=0.001000
  EtherCAT Rx Var 17 : xpcethercatlib/EtherCAT Rx Var   Priority=2  sig_name=Box 5 (ATRIAS 2.1 Hip (Medulla 1.5)).uController Status.ID  sig_offset=1968  sig_type=uint8  type_size=8  sig_dim=1  device_id=0  sample_time=0.001000
  EtherCAT Rx Var 18 : xpcethercatlib/EtherCAT Rx Var   Priority=2  sig_name=Box 5 (ATRIAS 2.1 Hip (Medulla 1.5)).uController Status.Limit Switch  sig_offset=2000  sig_type=uint8  type_size=8  sig_dim=1  device_id=0  sample_time=0.001000
  EtherCAT Rx Var 19 : xpcethercatlib/EtherCAT Rx Var   Priority=2  sig_name=Box 5 (ATRIAS 2.1 Hip (Medulla 1.5)).uController Status.State  sig_offset=1976  sig_type=uint8  type_size=8  sig_dim=1  device_id=0  sample_time=0.001000
  EtherCAT Rx Var 2 : xpcethercatlib/EtherCAT Rx Var   Priority=2  sig_name=Box 5 (ATRIAS 2.1 Hip (Medulla 1.5)).Incremental Encoder.Incremental Encoder  sig_offset=2152  sig_type=uint16  type_size=16  sig_dim=1  device_id=0  sample_time=0.001000
  EtherCAT Rx Var 3 : xpcethercatlib/EtherCAT Rx Var   Priority=2  sig_name=Box 5 (ATRIAS 2.1 Hip (Medulla 1.5)).Hip Encoder.Timestamp  sig_offset=2040  sig_type=uint16  type_size=16  sig_dim=1  device_id=0  sample_time=0.001000
  EtherCAT Rx Var 4 : xpcethercatlib/EtherCAT Rx Var   Priority=2  sig_name=Box 5 (ATRIAS 2.1 Hip (Medulla 1.5)).Hip Encoder.Encoder  sig_offset=2008  sig_type=uint32  type_size=32  sig_dim=1  device_id=0  sample_time=0.001000
  EtherCAT Rx Var 5 : xpcethercatlib/EtherCAT Rx Var   Priority=2  sig_name=Box 5 (ATRIAS 2.1 Hip (Medulla 1.5)).Incremental Encoder.Incremental Encoder Timestamp  sig_offset=2168  sig_type=uint16  type_size=16  sig_dim=1  device_id=0  sample_time=0.001000
  EtherCAT Rx Var 6 : xpcethercatlib/EtherCAT Rx Var   Priority=2  sig_name=Box 5 (ATRIAS 2.1 Hip (Medulla 1.5)).Power.Logic Voltage  sig_offset=2072  sig_type=uint16  type_size=16  sig_dim=1  device_id=0  sample_time=0.001000
  EtherCAT Tx Var 3 : xpcethercatlib/EtherCAT Tx Var   Priority=3  sig_name=Box 5 (ATRIAS 2.1 Hip (Medulla 1.5)).uControllerInput.Command  sig_offset=1968  sig_type=uint8  type_size=8  sig_dim=1  device_id=0  sample_time=0.001000
  EtherCAT Tx Var 4 : xpcethercatlib/EtherCAT Tx Var   Priority=3  sig_name=Box 5 (ATRIAS 2.1 Hip (Medulla 1.5)).uControllerInput.Counter  sig_offset=1976  sig_type=uint16  type_size=16  sig_dim=1  device_id=0  sample_time=0.001000
  EtherCAT Tx Var 5 : xpcethercatlib/EtherCAT Tx Var   Priority=3  sig_name=Box 5 (ATRIAS 2.1 Hip (Medulla 1.5)).uControllerInput.Motor Current  sig_offset=1992  sig_type=int32  type_size=32  sig_dim=1  device_id=0  sample_time=0.001000
  HipEncoder : Outport
  IncEncoder : Outport  Port=2
  LimitSwitch : Outport  Port=3
  ID : Outport  Port=4
  State : Outport  Port=5
  Counter : Outport  Port=6
  ErrorFlags : Outport  Port=7
  HipEncoderTimestamp : Outport  Port=8
  IncEncoderTimestamp : Outport  Port=9
  MotorVoltage : Outport  Port=10
  LogicVoltage : Outport  Port=11
  Thermistor0 : Outport  Port=12
  Thermistor1 : Outport  Port=13
  Thermistor2 : Outport  Port=14
  AmpMeasuredCurrent : Outport  Port=15
  wires:
  "EtherCAT Rx Var "/1 -> AmpMeasuredCurrent/1
  EtherCAT Rx Var 14/1 -> Thermistor2/1
  EtherCAT Rx Var 13/1 -> Thermistor1/1
  EtherCAT Rx Var 12/1 -> Thermistor0/1
  EtherCAT Rx Var 1/1 -> MotorVoltage/1
  EtherCAT Rx Var 6/1 -> LogicVoltage/1
  EtherCAT Rx Var 16/1 -> ErrorFlags/1
  EtherCAT Rx Var 19/1 -> State/1
  EtherCAT Rx Var 18/1 -> LimitSwitch/1
  EtherCAT Rx Var 17/1 -> ID/1
  EtherCAT Rx Var 15/1 -> Counter/1
  EtherCAT Rx Var 2/1 -> IncEncoder/1
  EtherCAT Rx Var 3/1 -> HipEncoderTimestamp/1
  EtherCAT Rx Var 4/1 -> HipEncoder/1
  EtherCAT Rx Var 5/1 -> IncEncoderTimestamp/1
  MotorCmd/1 -> Data Type Conversion5/1
  MedullaCounter/1 -> Data Type Conversion4/1
  MedullaCmd/1 -> Data Type Conversion3/1
  Data Type Conversion5/1 -> EtherCAT Tx Var 5/1
  Data Type Conversion4/1 -> EtherCAT Tx Var 4/1
  Data Type Conversion3/1 -> EtherCAT Tx Var 3/1

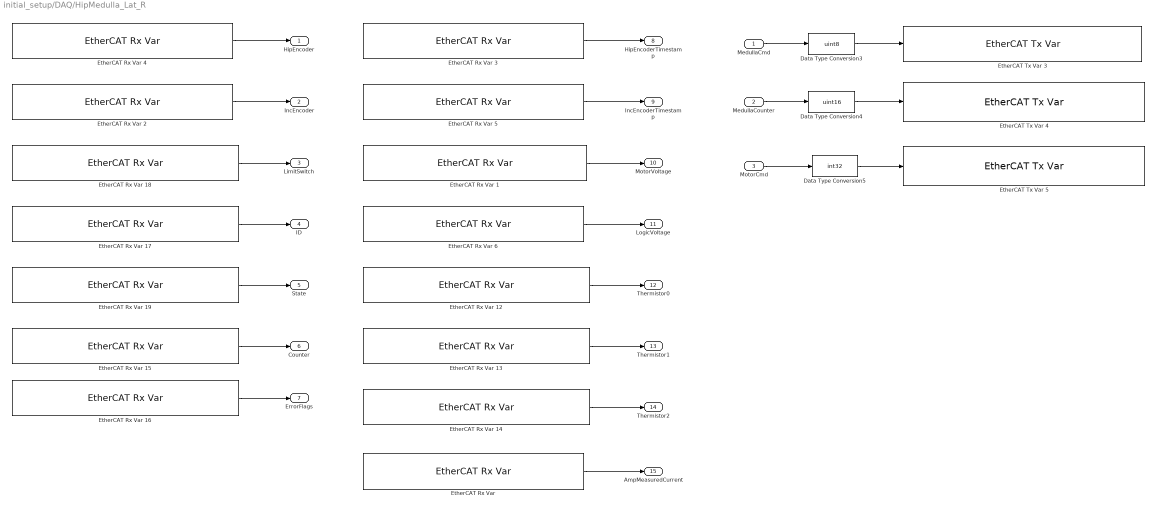
== system initial_setup/DAQ/HipMedulla_Lat_R ==
  MedullaCmd : Inport
  MedullaCounter : Inport  Port=2
  MotorCmd : Inport  Port=3
  Data Type Conversion3 : DataTypeConversion  OutDataTypeStr=uint8
  Data Type Conversion4 : DataTypeConversion  OutDataTypeStr=uint16
  Data Type Conversion5 : DataTypeConversion  OutDataTypeStr=int32
  "EtherCAT Rx Var " : xpcethercatlib/EtherCAT Rx Var   Priority=2  sig_name=Box 6 (ATRIAS 2.1 Hip (Medulla 1.5)).Measured Current.Amp Measured Current  sig_offset=2352  sig_type=int16  type_size=16  sig_dim=1  device_id=0  sample_time=0.001000
  EtherCAT Rx Var 1 : xpcethercatlib/EtherCAT Rx Var   Priority=2  sig_name=Box 6 (ATRIAS 2.1 Hip (Medulla 1.5)).Power.Motor Voltage  sig_offset=2272  sig_type=uint16  type_size=16  sig_dim=1  device_id=0  sample_time=0.001000
  EtherCAT Rx Var 12 : xpcethercatlib/EtherCAT Rx Var   Priority=2  sig_name=Box 6 (ATRIAS 2.1 Hip (Medulla 1.5)).Thermistors.Thermistor 0  sig_offset=2304  sig_type=uint16  type_size=16  sig_dim=1  device_id=0  sample_time=0.001000
  EtherCAT Rx Var 13 : xpcethercatlib/EtherCAT Rx Var   Priority=2  sig_name=Box 6 (ATRIAS 2.1 Hip (Medulla 1.5)).Thermistors.Thermistor 1  sig_offset=2320  sig_type=uint16  type_size=16  sig_dim=1  device_id=0  sample_time=0.001000
  EtherCAT Rx Var 14 : xpcethercatlib/EtherCAT Rx Var   Priority=2  sig_name=Box 6 (ATRIAS 2.1 Hip (Medulla 1.5)).Thermistors.Thermistor 2  sig_offset=2336  sig_type=uint16  type_size=16  sig_dim=1  device_id=0  sample_time=0.001000
  EtherCAT Rx Var 15 : xpcethercatlib/EtherCAT Rx Var   Priority=2  sig_name=Box 6 (ATRIAS 2.1 Hip (Medulla 1.5)).uController Status.Counter  sig_offset=2200  sig_type=uint8  type_size=8  sig_dim=1  device_id=0  sample_time=0.001000
  EtherCAT Rx Var 16 : xpcethercatlib/EtherCAT Rx Var   Priority=2  sig_name=Box 6 (ATRIAS 2.1 Hip (Medulla 1.5)).uController Status.Error Flags  sig_offset=2208  sig_type=uint8  type_size=8  sig_dim=1  device_id=0  sample_time=0.001000
  EtherCAT Rx Var 17 : xpcethercatlib/EtherCAT Rx Var   Priority=2  sig_name=Box 6 (ATRIAS 2.1 Hip (Medulla 1.5)).uController Status.ID  sig_offset=2184  sig_type=uint8  type_size=8  sig_dim=1  device_id=0  sample_time=0.001000
  EtherCAT Rx Var 18 : xpcethercatlib/EtherCAT Rx Var   Priority=2  sig_name=Box 6 (ATRIAS 2.1 Hip (Medulla 1.5)).uController Status.Limit Switch  sig_offset=2216  sig_type=uint8  type_size=8  sig_dim=1  device_id=0  sample_time=0.001000
  EtherCAT Rx Var 19 : xpcethercatlib/EtherCAT Rx Var   Priority=2  sig_name=Box 6 (ATRIAS 2.1 Hip (Medulla 1.5)).uController Status.State  sig_offset=2192  sig_type=uint8  type_size=8  sig_dim=1  device_id=0  sample_time=0.001000
  EtherCAT Rx Var 2 : xpcethercatlib/EtherCAT Rx Var   Priority=2  sig_name=Box 6 (ATRIAS 2.1 Hip (Medulla 1.5)).Incremental Encoder.Incremental Encoder  sig_offset=2368  sig_type=uint16  type_size=16  sig_dim=1  device_id=0  sample_time=0.001000
  EtherCAT Rx Var 3 : xpcethercatlib/EtherCAT Rx Var   Priority=2  sig_name=Box 6 (ATRIAS 2.1 Hip (Medulla 1.5)).Hip Encoder.Timestamp  sig_offset=2256  sig_type=uint16  type_size=16  sig_dim=1  device_id=0  sample_time=0.001000
  EtherCAT Rx Var 4 : xpcethercatlib/EtherCAT Rx Var   Priority=2  sig_name=Box 6 (ATRIAS 2.1 Hip (Medulla 1.5)).Hip Encoder.Encoder  sig_offset=2224  sig_type=uint32  type_size=32  sig_dim=1  device_id=0  sample_time=0.001000
  EtherCAT Rx Var 5 : xpcethercatlib/EtherCAT Rx Var   Priority=2  sig_name=Box 6 (ATRIAS 2.1 Hip (Medulla 1.5)).Incremental Encoder.Incremental Encoder Timestamp  sig_offset=2384  sig_type=uint16  type_size=16  sig_dim=1  device_id=0  sample_time=0.001000
  EtherCAT Rx Var 6 : xpcethercatlib/EtherCAT Rx Var   Priority=2  sig_name=Box 6 (ATRIAS 2.1 Hip (Medulla 1.5)).Power.Logic Voltage  sig_offset=2288  sig_type=uint16  type_size=16  sig_dim=1  device_id=0  sample_time=0.001000
  EtherCAT Tx Var 3 : xpcethercatlib/EtherCAT Tx Var   Priority=3  sig_name=Box 6 (ATRIAS 2.1 Hip (Medulla 1.5)).uControllerInput.Command  sig_offset=2184  sig_type=uint8  type_size=8  sig_dim=1  device_id=0  sample_time=0.001000
  EtherCAT Tx Var 4 : xpcethercatlib/EtherCAT Tx Var   Priority=3  sig_name=Box 6 (ATRIAS 2.1 Hip (Medulla 1.5)).uControllerInput.Counter  sig_offset=2192  sig_type=uint16  type_size=16  sig_dim=1  device_id=0  sample_time=0.001000
  EtherCAT Tx Var 5 : xpcethercatlib/EtherCAT Tx Var   Priority=3  sig_name=Box 6 (ATRIAS 2.1 Hip (Medulla 1.5)).uControllerInput.Motor Current  sig_offset=2208  sig_type=int32  type_size=32  sig_dim=1  device_id=0  sample_time=0.001000
  HipEncoder : Outport
  IncEncoder : Outport  Port=2
  LimitSwitch : Outport  Port=3
  ID : Outport  Port=4
  State : Outport  Port=5
  Counter : Outport  Port=6
  ErrorFlags : Outport  Port=7
  HipEncoderTimestamp : Outport  Port=8
  IncEncoderTimestamp : Outport  Port=9
  MotorVoltage : Outport  Port=10
  LogicVoltage : Outport  Port=11
  Thermistor0 : Outport  Port=12
  Thermistor1 : Outport  Port=13
  Thermistor2 : Outport  Port=14
  AmpMeasuredCurrent : Outport  Port=15
  wires:
  "EtherCAT Rx Var "/1 -> AmpMeasuredCurrent/1
  EtherCAT Rx Var 14/1 -> Thermistor2/1
  EtherCAT Rx Var 13/1 -> Thermistor1/1
  EtherCAT Rx Var 12/1 -> Thermistor0/1
  EtherCAT Rx Var 1/1 -> MotorVoltage/1
  EtherCAT Rx Var 6/1 -> LogicVoltage/1
  EtherCAT Rx Var 16/1 -> ErrorFlags/1
  EtherCAT Rx Var 19/1 -> State/1
  EtherCAT Rx Var 18/1 -> LimitSwitch/1
  EtherCAT Rx Var 17/1 -> ID/1
  EtherCAT Rx Var 15/1 -> Counter/1
  EtherCAT Rx Var 2/1 -> IncEncoder/1
  EtherCAT Rx Var 3/1 -> HipEncoderTimestamp/1
  EtherCAT Rx Var 4/1 -> HipEncoder/1
  EtherCAT Rx Var 5/1 -> IncEncoderTimestamp/1
  MotorCmd/1 -> Data Type Conversion5/1
  MedullaCounter/1 -> Data Type Conversion4/1
  MedullaCmd/1 -> Data Type Conversion3/1
  Data Type Conversion5/1 -> EtherCAT Tx Var 5/1
  Data Type Conversion4/1 -> EtherCAT Tx Var 4/1
  Data Type Conversion3/1 -> EtherCAT Tx Var 3/1
